simulink model "untitled1"  (R2023a)
settings: Solver=VariableStepAuto  StartTime=0.0  StopTime=10.0  RelTol=1e-3
settings Model: Creator=huang  LastModifiedBy=huang

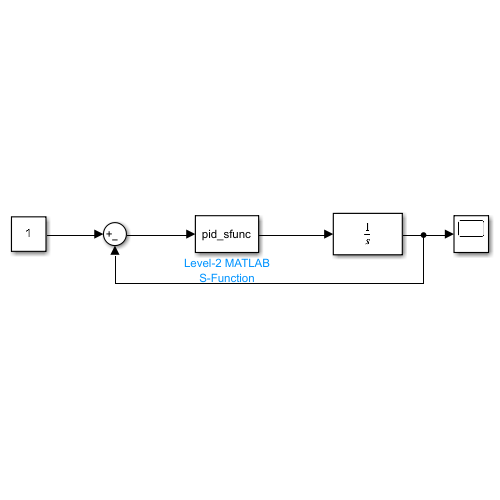
[thumbnail: Simulink's stored preview of the top-level diagram]
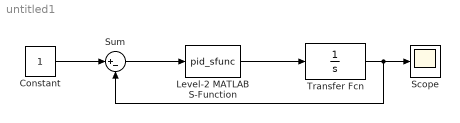
== system untitled1 ==
  Constant : Constant
  Level-2 MATLAB S-Function : M-S-Function  FunctionName=pid_sfunc
  Scope : Scope
  Sum : Sum  Inputs=|+-
  Transfer Fcn : TransferFcn  Denominator=[1 0]
  wires:
  Constant/1 -> Sum/1
  Sum/1 -> Level-2 MATLAB S-Function/1
  Transfer Fcn/1 -> Sum/2, Scope/1
  Level-2 MATLAB S-Function/1 -> Transfer Fcn/1
